simulink model "mpc_bogko"  (R2024b)
settings: Solver=VariableStepAuto  StartTime=0.0  StopTime=10  FixedStep=0.01  RelTol=1e-3
model workspace (MAT data in the model file):
  AlgnTrqCambCompl = [0 0 0 0]
  AlgnTrqSteerCompl = [0 0 0 0]
  AxlIxx = 62.3745166667
  AxlM = 160
  BumpCamber = [0 0 0 0]
  BumpCaster = [0 0 0 0]
  BumpSteer = [0 0 0 0]
  CambVsSteerAng = [0 0 0 0]
  CastVsSteerAng = [0 0 0 0]
  Cps = 2
  Cz = 5565.2246438
  CzWhlAxl = 11490.971257
  DCT_Param : object (value not decoded)
  DLCXref = [0 6.1 6.2 18 33 33.5 45 50 60]
  DLCXrefStanley1 = [0 2.4 4.8 7.2 9.6 12 17.2002368196 22.3752654753 27.5 32.6247345247 37.7997631804 43 ... (32 elements, 1x32)]
  DLCXrefStanley2 = [0 1.2 2.4 3.6 4.8 6 7.2 8.4 9.44987166868 10.0991210544 10.1 10.1008789456 ... (38 elements, 1x38)]
  DLCYref = [0 0 -5 -3.875 -3.5 1 0 0 0]
  DLCYrefStanley1 = [0 0 0 0 0 0 -0.181140468595 -0.723683795406 -1.625 -2.52631620459 -3.0688595314 -3.25 ... (32 elements, 1x32)]
  DLCYrefStanley2 = [0.1375 0.1375 0.1375 0.1375 0.1375 0.1375 0.1375 0.1375 -0.203439148031 -1.09615705337 -2.2 -3.30384294663 ... (38 elements, 1x38)]
  Downshift_Speeds = [9.5625 12.9375 16.3125 19.6875 23.0625 26.4375 29.8125 33.1875 36.5625 39.9375 43.3125 46.6875 ... (28 elements, 4x7)]
  EngRevLim = 7000
  F0z = [1067 933]
  F0zWhlAxl = 2907
  Hmax = 0.25
  Kz = 52451.0065793
  KzWhlAxl = 138031.612078
  LatCambCompl = [0 0 0 0]
  LatSteerCompl = [0 0 0 0]
  LatWhlCtrComplLat = [0 0 0 0]
  LatWhlCtrComplLngBrk = [0  0  0  0; 0  0  0  0]
  LatWhlCtrDisp = [0 0 0 0]
  LngCambCompl = [0  0  0  0; 0  0  0  0]
  LngCastCompl = [0  0  0  0; 0  0  0  0]
  LngSteerCompl = [0  0  0  0; 0  0  0  0]
  LngWhlCtrCompl = [0  0  0  0; 0  0  0  0]
  LngWhlCtrDisp = [0 0 0 0]
  MotRatios = [1 1]
  NCyl = 6
  NrmlWhlFrcOff = [2886 2886 2907 2907]
  NrmlWhlRates = [52.4510065793 52.4510065793 52.4510065793 52.4510065793]
  Pedal_Positions = [0.1 0.4 0.5 0.9]
  Pstd = 101325
  Rair = 287
  RollCamber : object (value not decoded)
  RollCaster : object (value not decoded)
  RollSteer : object (value not decoded)
  RollStiffArb = [0 0]
  RollStiffArbFrnt = 800
  RollStiffNoArb = [0 0]
  RollStiffNoArbFrnt = 0
  RollStiffNoTwstRear = 0
  ShckFrcVsCompRate = [5.5652246438 5.5652246438 5.5652246438 5.5652246438]
  Sig : Simulink.Signal (value not decoded)
  Sig1 : Simulink.Signal (value not decoded)
  StatCamber = [0 0 0 0]
  StatCaster = [0 0 0 0]
  StatLdWhlR = [0.3 0.3 0.3 0.3]
  StatToe = [0 0 0 0]
  Trans : object (value not decoded)
  Tstd = 293.15
  Upshift_Speeds = [12.9375 16.3125 19.6875 33 26.4375 29.8125 33.1875 52.5 39.9375 43.3125 46.6875 77.25 ... (28 elements, 4x7)]
  VEH : object (value not decoded)
  Vd = 0.00346
  VrtLdTrnsfr = [0 0 0 0]
  WH : Mass (value not decoded)
  dt3D = 0.05
  f_air = [0 0 0 0 0 0 0 0 0 0 0 0 ... (256 elements, 16x16)]
  f_co = [0 0 0 0 0 0 0 0 0 0 0 0 ... (256 elements, 16x16)]
  f_co2 = [0 0 0 0 0 0 0 0 0 0 0 0 ... (256 elements, 16x16)]
  f_eff = [352.135682859 352.135682859 320.724378192 303.655312657 295.930136708 291.240087194 291.240271258 291.240312459 291.240275452 291.240198499 291.240100781 291.240018769 ... (256 elements, 16x16)]
  f_fuel = [0 0 0 0 0 0 0 0 0 0 0 0 ... (256 elements, 16x16)]
  f_hc = [0 0 0 0 0 0 0 0 0 0 0 0 ... (256 elements, 16x16)]
  f_nox = [0 0 0 0 0 0 0 0 0 0 0 0 ... (256 elements, 16x16)]
  f_pm = [0 0 0 0 0 0 0 0 0 0 0 0 ... (256 elements, 16x16)]
  f_susp_axl_bp = [1 2]
  f_susp_dz_bp = [-0.325022776267 -0.315022776267 -0.305022776267 -0.205022776267 -0.105022776267 -0.00502277626717 0.0949772237328 0.194977223733 0.204977223733 0.214977223733]
  f_susp_dzdot_bp = [-3 -0.3 -0.2 -0.1 0 0.1 0.2 0.3 3]
  f_susp_fmz = [-144070.391448 -93629.24037 -75929.1118915 -20630.5828179 -15385.48216 -10140.3815021 -4895.28084414 349.819813785 -31916.3973792 18437.6709544 -83996.1993354 -33555.0482577 ... (43920 elements, 10x9x61x2x4)]
  f_susp_geom = [0 0 0 0 0 0 0 0 0 0 0 0 ... (3660 elements, 10x61x2x3)]
  f_susp_strgdelta_bp = [-0.523598775598 -0.506145483078 -0.488692190558 -0.471238898038 -0.453785605519 -0.436332312999 -0.418879020479 -0.401425727959 -0.383972435439 -0.366519142919 -0.349065850399 -0.331612557879 ... (61 elements, 1x61)]
  f_tbrake = [0 76.8593923996 105.140482948 131.533638111 157.926793274 176.658631717 176.65727296 176.656856686 176.656879077 176.657093756 176.657404516 176.65772406 ... (256 elements, 16x16)]
  f_tbrake_n_bpt = [0 649.519052838 912.419621844 1175.32019085 1438.22075986 1701.12132886 1964.02189787 2226.92246687 2489.82303588 2752.72360489 3015.62417389 3278.5247429 ... (16 elements, 1x16)]
  f_tbrake_t_bpt = [0 34.6410161514 61.0341713143 87.4273264773 113.82048164 140.213636803 166.606791966 192.999947129 219.393102292 245.786257455 272.179412618 298.572567781 ... (16 elements, 1x16)]
  f_texh = [766.752464599 766.752464599 786.17542386 801.679939032 884.591982581 910.574397722 910.571871054 910.570774534 910.570601632 910.570821151 910.571247242 910.571639815 ... (256 elements, 16x16)]
  f_twc_eff_co = [0.17 0.25 0.45 0.99 0.99 0.99 0.99]
  f_twc_eff_hc = [0.21 0.375 0.75 0.98 0.98 0.98 0.98]
  f_twc_eff_lam = [0.909090909 0.944055944 0.979020979 1 1.013986014 1.048951049 1.083916084]
  f_twc_eff_nox = [0.98 0.98 0.98 0.97 0.05 0.02 0]
  numWheel = 4
  rayDirections = [0 0 0 0 0 0 0 0 0 0 0 0 ... (363 elements, 121x3)]
  rayLengths = [20 20 20 20 20 20 20 20 20 20 20 20 ... (121 elements, 121x1)]
  rayOrigins = [0.5 0.4 0.3 0.2 0.1 0 -0.1 -0.2 -0.3 -0.4 -0.5 0.5 ... (363 elements, 121x3)]
values from neighbouring files (symbols this model uses):
  a = -2*(Cf+Cr)/(m*V)    (= -1.53333333333)    [continuousDynamics.m]    (also in getting_lqr_gain.m = -1.91273333333; mpc_simulation.m; road.m = 1.4)
  b = -1-2*(Cf*Lf-Cr*Lr)/(m*V^2)    (= -0.996444444444)    [continuousDynamics.m]    (also in getting_lqr_gain.m = -0.976308444444; mpc_simulation.m; road.m = 1.6)
  beta_road = road(:,4)    [analytic_simulation.m]    (also in lqr_simulation.m; mpc_simulation.m; plotting.m)
  c = -2*((Cf*Lf-Cr*Lr)/Jz)    (= 0.4)    [continuousDynamics.m]    (also in getting_lqr_gain.m = 2.6653; mpc_simulation.m)
  D = [0]    [getting_lqr_gain.m]    (also in mpc_simulation.m = zeros(nx,1))
  t_road = road(:,1)    [analytic_simulation.m]    (also in lqr_simulation.m; mpc_simulation.m; plotting.m; road.m = 0:dt:t_end)
  yaw_rate_road = road(:,5)    [analytic_simulation.m]    (also in lqr_simulation.m; mpc_simulation.m)
symbols that are objects in the model workspace (value not decoded): VEH
libraries: vehdynlibtire x11, vehdynlibsuspension x8, sharedtransform x6, autolibutils x5, instrumentseriallib x3, sim3dgroundtruthsensorlib x2, SignalEditorBlockLib x2, shared6dof x2, svdutilitieslib x1, vehdynlibviscommon x1, vehdynlibsteering x1, hdlsllib x1
(part 9 of 9)

== system mpc_bogko/Vehicle/Variant Subsystem/6DOF/Suspension to Chasiss Transforms/Susp2Body ==
  DCM : Inport
  VehAng : Inport  Port=2
  SuspAng : Inport  Port=3
  Fs : Inport  Port=4  Partition=on  PartitionDimension=2  PartitionWidth=1  PartitionOffset=0
  Ms : Inport  Port=5  Partition=on  PartitionDimension=2  PartitionWidth=1  PartitionOffset=0
  For Each : ForEach  DisableCoverage=on
  Inertial to Body : Product  Multiplication=Matrix(*)  InputSameDT=on  SaturateOnIntegerOverflow=on  OutDataTypeStr=Inherit: Same as first input
  Inertial to Body1 : Product  Multiplication=Matrix(*)  InputSameDT=on  SaturateOnIntegerOverflow=on  OutDataTypeStr=Inherit: Same as first input
  Reshape : Reshape
  Reshape1 : Reshape
  Rotation Angles to Direction Cosine Matrix : sharedtransform/Rotation Angles to Direction Cosine Matrix  rotationOrder=ZYX  aMode=2
  Selector : Selector  InputPortWidth=3  IndexOptions=Index vector (dialog)  Indices=[3 2 1]  OutputSizes=1
  Selector1 : Selector  InputPortWidth=3  IndexOptions=Index vector (dialog)  Indices=[1 2]  OutputSizes=1
  Selector2 : Selector  InputPortWidth=3  IndexOptions=Index vector (dialog)  Indices=[3]  OutputSizes=1
  Transpose : Math  Operator=transpose  SignedPower=on
  Unary Minus : UnaryMinus
  Vector Concatenate : Concatenate
  "transform to Inertial axes " : shared6dof/6DOF (Euler Angles)/transform to Inertial axes   SystemSampleTime=-1  VariantActivationTime=update diagram  AllowFlexibleInterface=on  Latency=0  AutoFrameSizeCalculation=off
  transform to Inertial axes 1 : shared6dof/6DOF (Euler Angles)/transform to Inertial axes   SystemSampleTime=-1  VariantActivationTime=update diagram  AllowFlexibleInterface=on  Latency=0  AutoFrameSizeCalculation=off
  FsB : Outport  ConcatenationDimension=2  VectorParamsAs1DForOutWhenUnconnected=off
  MsB : Outport  Port=2  ConcatenationDimension=2  VectorParamsAs1DForOutWhenUnconnected=off
  wires:
  Reshape/1 -> Inertial to Body/2
  Inertial to Body/1 -> FsB/1
  SuspAng/1 -> Unary Minus/1
  Selector/1 -> Rotation Angles to Direction Cosine Matrix/1
  Fs/1 -> "transform to Inertial axes "/1
  Transpose/1 -> transform to Inertial axes 1/2, "transform to Inertial axes "/2
  Rotation Angles to Direction Cosine Matrix/1 -> Transpose/1
  "transform to Inertial axes "/1 -> Reshape/1
  transform to Inertial axes 1/1 -> Reshape1/1
  Inertial to Body1/1 -> MsB/1
  Reshape1/1 -> Inertial to Body1/2
  DCM/1 -> Inertial to Body1/1, Inertial to Body/1
  Ms/1 -> transform to Inertial axes 1/1
  VehAng/1 -> Selector2/1
  Unary Minus/1 -> Selector1/1
  Selector1/1 -> Vector Concatenate/1
  Vector Concatenate/1 -> Selector/1
  Selector2/1 -> Vector Concatenate/2

== system mpc_bogko/Wheels and Tires/VDBS/Tires/Fiala Tires/Fx ==
  In1 : Inport
  In2 : Inport  Port=2
  In3 : Inport  Port=3
  In4 : Inport  Port=4
  Bus Selector{,1..3} (4 alike) : BusSelector  OutputSignals=Fx
  Vector Concatenate : Concatenate  NumInputs=4
  Out1 : Outport  VectorParamsAs1DForOutWhenUnconnected=off
  wires:
  Bus Selector3/1 -> Vector Concatenate/4  "<Fx>"
  Bus Selector2/1 -> Vector Concatenate/3  "<Fx>"
  Bus Selector1/1 -> Vector Concatenate/2  "<Fx>"
  In4/1 -> Bus Selector3/1
  In3/1 -> Bus Selector2/1
  In2/1 -> Bus Selector1/1
  Bus Selector/1 -> Vector Concatenate/1  "<Fx>"
  In1/1 -> Bus Selector/1
  Vector Concatenate/1 -> Out1/1

== system mpc_bogko/Wheels and Tires/VDBS/Tires/Fiala Tires/Fy ==
  In1 : Inport
  In2 : Inport  Port=2
  In3 : Inport  Port=3
  In4 : Inport  Port=4
  Bus Selector{,1..3} (4 alike) : BusSelector  OutputSignals=Fy
  Vector Concatenate : Concatenate  NumInputs=4
  Out1 : Outport  VectorParamsAs1DForOutWhenUnconnected=off
  wires:
  Vector Concatenate/1 -> Out1/1
  In1/1 -> Bus Selector/1
  Bus Selector/1 -> Vector Concatenate/1  "<Fy>"
  In2/1 -> Bus Selector1/1
  In3/1 -> Bus Selector2/1
  In4/1 -> Bus Selector3/1
  Bus Selector1/1 -> Vector Concatenate/2  "<Fy>"
  Bus Selector2/1 -> Vector Concatenate/3  "<Fy>"
  Bus Selector3/1 -> Vector Concatenate/4  "<Fy>"

== system mpc_bogko/Wheels and Tires/VDBS/Tires/Fiala Tires/Fz ==
  In1 : Inport
  In2 : Inport  Port=2
  In3 : Inport  Port=3
  In4 : Inport  Port=4
  Bus Selector{,1..3} (4 alike) : BusSelector  OutputSignals=Fz
  Vector Concatenate : Concatenate  NumInputs=4
  Out1 : Outport  VectorParamsAs1DForOutWhenUnconnected=off
  wires:
  Vector Concatenate/1 -> Out1/1
  In1/1 -> Bus Selector/1
  Bus Selector/1 -> Vector Concatenate/1  "<Fz>"
  In2/1 -> Bus Selector1/1
  In3/1 -> Bus Selector2/1
  In4/1 -> Bus Selector3/1
  Bus Selector1/1 -> Vector Concatenate/2  "<Fz>"
  Bus Selector2/1 -> Vector Concatenate/3  "<Fz>"
  Bus Selector3/1 -> Vector Concatenate/4  "<Fz>"

== system mpc_bogko/Wheels and Tires/VDBS/Tires/Fiala Tires/Mx ==
  In1 : Inport
  In2 : Inport  Port=2
  In3 : Inport  Port=3
  In4 : Inport  Port=4
  Bus Selector{,1..3} (4 alike) : BusSelector  OutputSignals=Mx
  Vector Concatenate : Concatenate  NumInputs=4
  Out1 : Outport  VectorParamsAs1DForOutWhenUnconnected=off
  wires:
  Vector Concatenate/1 -> Out1/1
  In1/1 -> Bus Selector/1
  Bus Selector/1 -> Vector Concatenate/1  "<Mx>"
  In2/1 -> Bus Selector1/1
  In3/1 -> Bus Selector2/1
  In4/1 -> Bus Selector3/1
  Bus Selector1/1 -> Vector Concatenate/2  "<Mx>"
  Bus Selector2/1 -> Vector Concatenate/3  "<Mx>"
  Bus Selector3/1 -> Vector Concatenate/4  "<Mx>"

== system mpc_bogko/Wheels and Tires/VDBS/Tires/Fiala Tires/My ==
  In1 : Inport
  In2 : Inport  Port=2
  In3 : Inport  Port=3
  In4 : Inport  Port=4
  Bus Selector{,1..3} (4 alike) : BusSelector  OutputSignals=My
  Vector Concatenate : Concatenate  NumInputs=4
  Out1 : Outport  VectorParamsAs1DForOutWhenUnconnected=off
  wires:
  Bus Selector3/1 -> Vector Concatenate/4  "<My>"
  Bus Selector2/1 -> Vector Concatenate/3  "<My>"
  Bus Selector1/1 -> Vector Concatenate/2  "<My>"
  In4/1 -> Bus Selector3/1
  In3/1 -> Bus Selector2/1
  In2/1 -> Bus Selector1/1
  Bus Selector/1 -> Vector Concatenate/1  "<My>"
  In1/1 -> Bus Selector/1
  Vector Concatenate/1 -> Out1/1

== system mpc_bogko/Wheels and Tires/VDBS/Tires/Fiala Tires/Mz ==
  In1 : Inport
  In2 : Inport  Port=2
  In3 : Inport  Port=3
  In4 : Inport  Port=4
  Bus Selector{,1..3} (4 alike) : BusSelector  OutputSignals=Mz
  Vector Concatenate : Concatenate  NumInputs=4
  Out1 : Outport  VectorParamsAs1DForOutWhenUnconnected=off
  wires:
  Bus Selector3/1 -> Vector Concatenate/4  "<Mz>"
  Bus Selector2/1 -> Vector Concatenate/3  "<Mz>"
  Bus Selector1/1 -> Vector Concatenate/2  "<Mz>"
  In4/1 -> Bus Selector3/1
  In3/1 -> Bus Selector2/1
  In2/1 -> Bus Selector1/1
  Bus Selector/1 -> Vector Concatenate/1  "<Mz>"
  In1/1 -> Bus Selector/1
  Vector Concatenate/1 -> Out1/1

== system mpc_bogko/Wheels and Tires/VDBS/Tires/Fiala Tires/Re ==
  In1 : Inport
  In2 : Inport  Port=2
  In3 : Inport  Port=3
  In4 : Inport  Port=4
  Bus Selector{,1..3} (4 alike) : BusSelector  OutputSignals=Re
  Vector Concatenate : Concatenate  NumInputs=4
  Out1 : Outport  VectorParamsAs1DForOutWhenUnconnected=off
  wires:
  Vector Concatenate/1 -> Out1/1
  In1/1 -> Bus Selector/1
  Bus Selector/1 -> Vector Concatenate/1  "<Re>"
  In2/1 -> Bus Selector1/1
  In3/1 -> Bus Selector2/1
  In4/1 -> Bus Selector3/1
  Bus Selector1/1 -> Vector Concatenate/2  "<Re>"
  Bus Selector2/1 -> Vector Concatenate/3  "<Re>"
  Bus Selector3/1 -> Vector Concatenate/4  "<Re>"

== system mpc_bogko/Wheels and Tires/VDBS/Tires/Fiala Tires/alpha ==
  In1 : Inport
  In2 : Inport  Port=2
  In3 : Inport  Port=3
  In4 : Inport  Port=4
  Bus Selector{,1..3} (4 alike) : BusSelector  OutputSignals=Alpha
  Vector Concatenate : Concatenate  NumInputs=4
  Out1 : Outport  VectorParamsAs1DForOutWhenUnconnected=off
  wires:
  Vector Concatenate/1 -> Out1/1
  In1/1 -> Bus Selector/1
  Bus Selector/1 -> Vector Concatenate/1  "<Alpha>"
  In2/1 -> Bus Selector1/1
  In3/1 -> Bus Selector2/1
  In4/1 -> Bus Selector3/1
  Bus Selector1/1 -> Vector Concatenate/2  "<Alpha>"
  Bus Selector2/1 -> Vector Concatenate/3  "<Alpha>"
  Bus Selector3/1 -> Vector Concatenate/4  "<Alpha>"

== system mpc_bogko/Wheels and Tires/VDBS/Tires/Fiala Tires/kappa ==
  In1 : Inport
  In2 : Inport  Port=2
  In3 : Inport  Port=3
  In4 : Inport  Port=4
  Bus Selector{,1..3} (4 alike) : BusSelector  OutputSignals=Kappa
  Vector Concatenate : Concatenate  NumInputs=4
  Out1 : Outport  VectorParamsAs1DForOutWhenUnconnected=off
  wires:
  Bus Selector3/1 -> Vector Concatenate/4  "<Kappa>"
  Bus Selector2/1 -> Vector Concatenate/3  "<Kappa>"
  Bus Selector1/1 -> Vector Concatenate/2  "<Kappa>"
  In4/1 -> Bus Selector3/1
  In3/1 -> Bus Selector2/1
  In2/1 -> Bus Selector1/1
  Bus Selector/1 -> Vector Concatenate/1  "<Kappa>"
  In1/1 -> Bus Selector/1
  Vector Concatenate/1 -> Out1/1

== system mpc_bogko/Wheels and Tires/VDBS/Tires/Fiala Tires/omega ==
  In1 : Inport
  In2 : Inport  Port=2
  In3 : Inport  Port=3
  In4 : Inport  Port=4
  Bus Selector{,1..3} (4 alike) : BusSelector  OutputSignals=Omega
  Vector Concatenate : Concatenate  NumInputs=4
  Out1 : Outport  VectorParamsAs1DForOutWhenUnconnected=off
  wires:
  In1/1 -> Bus Selector/1
  Bus Selector/1 -> Vector Concatenate/1  "<Omega>"
  In2/1 -> Bus Selector1/1
  In3/1 -> Bus Selector2/1
  In4/1 -> Bus Selector3/1
  Bus Selector1/1 -> Vector Concatenate/2  "<Omega>"
  Bus Selector2/1 -> Vector Concatenate/3  "<Omega>"
  Bus Selector3/1 -> Vector Concatenate/4  "<Omega>"
  Vector Concatenate/1 -> Out1/1

== system mpc_bogko/Wheels and Tires/VDBS/Tires/Fiala Tires/z ==
  In1 : Inport
  In2 : Inport  Port=2
  In3 : Inport  Port=3
  In4 : Inport  Port=4
  Bus Selector{,1..3} (4 alike) : BusSelector  OutputSignals=z
  Vector Concatenate : Concatenate  NumInputs=4
  Out1 : Outport  VectorParamsAs1DForOutWhenUnconnected=off
  wires:
  Bus Selector3/1 -> Vector Concatenate/4  "<z>"
  Bus Selector2/1 -> Vector Concatenate/3  "<z>"
  Bus Selector1/1 -> Vector Concatenate/2  "<z>"
  In4/1 -> Bus Selector3/1
  In3/1 -> Bus Selector2/1
  In2/1 -> Bus Selector1/1
  Bus Selector/1 -> Vector Concatenate/1  "<z>"
  In1/1 -> Bus Selector/1
  Vector Concatenate/1 -> Out1/1

== system mpc_bogko/Wheels and Tires/VDBS/Tires/Fiala Tires/zdot ==
  In1 : Inport
  In2 : Inport  Port=2
  In3 : Inport  Port=3
  In4 : Inport  Port=4
  Bus Selector{,1..3} (4 alike) : BusSelector  OutputSignals=zdot
  Vector Concatenate : Concatenate  NumInputs=4
  Out1 : Outport  VectorParamsAs1DForOutWhenUnconnected=off
  wires:
  Vector Concatenate/1 -> Out1/1
  In1/1 -> Bus Selector/1
  Bus Selector/1 -> Vector Concatenate/1  "<zdot>"
  In2/1 -> Bus Selector1/1
  In3/1 -> Bus Selector2/1
  In4/1 -> Bus Selector3/1
  Bus Selector1/1 -> Vector Concatenate/2  "<zdot>"
  Bus Selector2/1 -> Vector Concatenate/3  "<zdot>"
  Bus Selector3/1 -> Vector Concatenate/4  "<zdot>"

== system mpc_bogko/Wheels and Tires/VDBS/Tires/MF Tires/Fx ==
  In1 : Inport
  In2 : Inport  Port=2
  In3 : Inport  Port=3
  In4 : Inport  Port=4
  Bus Selector{,1..3} (4 alike) : BusSelector  OutputSignals=Fx
  Vector Concatenate : Concatenate  NumInputs=4
  Out1 : Outport  VectorParamsAs1DForOutWhenUnconnected=off
  wires:
  Bus Selector3/1 -> Vector Concatenate/4  "<Fx>"
  Bus Selector2/1 -> Vector Concatenate/3  "<Fx>"
  Bus Selector1/1 -> Vector Concatenate/2  "<Fx>"
  In4/1 -> Bus Selector3/1
  In3/1 -> Bus Selector2/1
  In2/1 -> Bus Selector1/1
  Bus Selector/1 -> Vector Concatenate/1  "<Fx>"
  In1/1 -> Bus Selector/1
  Vector Concatenate/1 -> Out1/1

== system mpc_bogko/Wheels and Tires/VDBS/Tires/MF Tires/Fy ==
  In1 : Inport
  In2 : Inport  Port=2
  In3 : Inport  Port=3
  In4 : Inport  Port=4
  Bus Selector{,1..3} (4 alike) : BusSelector  OutputSignals=Fy
  Vector Concatenate : Concatenate  NumInputs=4
  Out1 : Outport  VectorParamsAs1DForOutWhenUnconnected=off
  wires:
  Vector Concatenate/1 -> Out1/1
  In1/1 -> Bus Selector/1
  Bus Selector/1 -> Vector Concatenate/1  "<Fy>"
  In2/1 -> Bus Selector1/1
  In3/1 -> Bus Selector2/1
  In4/1 -> Bus Selector3/1
  Bus Selector1/1 -> Vector Concatenate/2  "<Fy>"
  Bus Selector2/1 -> Vector Concatenate/3  "<Fy>"
  Bus Selector3/1 -> Vector Concatenate/4  "<Fy>"

== system mpc_bogko/Wheels and Tires/VDBS/Tires/MF Tires/Fz ==
  In1 : Inport
  In2 : Inport  Port=2
  In3 : Inport  Port=3
  In4 : Inport  Port=4
  Bus Selector{,1..3} (4 alike) : BusSelector  OutputSignals=Fz
  Vector Concatenate : Concatenate  NumInputs=4
  Out1 : Outport  VectorParamsAs1DForOutWhenUnconnected=off
  wires:
  Vector Concatenate/1 -> Out1/1
  In1/1 -> Bus Selector/1
  Bus Selector/1 -> Vector Concatenate/1  "<Fz>"
  In2/1 -> Bus Selector1/1
  In3/1 -> Bus Selector2/1
  In4/1 -> Bus Selector3/1
  Bus Selector1/1 -> Vector Concatenate/2  "<Fz>"
  Bus Selector2/1 -> Vector Concatenate/3  "<Fz>"
  Bus Selector3/1 -> Vector Concatenate/4  "<Fz>"

== system mpc_bogko/Wheels and Tires/VDBS/Tires/MF Tires/Mx ==
  In1 : Inport
  In2 : Inport  Port=2
  In3 : Inport  Port=3
  In4 : Inport  Port=4
  Bus Selector{,1..3} (4 alike) : BusSelector  OutputSignals=Mx
  Vector Concatenate : Concatenate  NumInputs=4
  Out1 : Outport  VectorParamsAs1DForOutWhenUnconnected=off
  wires:
  Vector Concatenate/1 -> Out1/1
  In1/1 -> Bus Selector/1
  Bus Selector/1 -> Vector Concatenate/1  "<Mx>"
  In2/1 -> Bus Selector1/1
  In3/1 -> Bus Selector2/1
  In4/1 -> Bus Selector3/1
  Bus Selector1/1 -> Vector Concatenate/2  "<Mx>"
  Bus Selector2/1 -> Vector Concatenate/3  "<Mx>"
  Bus Selector3/1 -> Vector Concatenate/4  "<Mx>"

== system mpc_bogko/Wheels and Tires/VDBS/Tires/MF Tires/My ==
  In1 : Inport
  In2 : Inport  Port=2
  In3 : Inport  Port=3
  In4 : Inport  Port=4
  Bus Selector{,1..3} (4 alike) : BusSelector  OutputSignals=My
  Vector Concatenate : Concatenate  NumInputs=4
  Out1 : Outport  VectorParamsAs1DForOutWhenUnconnected=off
  wires:
  Bus Selector3/1 -> Vector Concatenate/4  "<My>"
  Bus Selector2/1 -> Vector Concatenate/3  "<My>"
  Bus Selector1/1 -> Vector Concatenate/2  "<My>"
  In4/1 -> Bus Selector3/1
  In3/1 -> Bus Selector2/1
  In2/1 -> Bus Selector1/1
  Bus Selector/1 -> Vector Concatenate/1  "<My>"
  In1/1 -> Bus Selector/1
  Vector Concatenate/1 -> Out1/1

== system mpc_bogko/Wheels and Tires/VDBS/Tires/MF Tires/Mz ==
  In1 : Inport
  In2 : Inport  Port=2
  In3 : Inport  Port=3
  In4 : Inport  Port=4
  Bus Selector{,1..3} (4 alike) : BusSelector  OutputSignals=Mz
  Vector Concatenate : Concatenate  NumInputs=4
  Out1 : Outport  VectorParamsAs1DForOutWhenUnconnected=off
  wires:
  Bus Selector3/1 -> Vector Concatenate/4  "<Mz>"
  Bus Selector2/1 -> Vector Concatenate/3  "<Mz>"
  Bus Selector1/1 -> Vector Concatenate/2  "<Mz>"
  In4/1 -> Bus Selector3/1
  In3/1 -> Bus Selector2/1
  In2/1 -> Bus Selector1/1
  Bus Selector/1 -> Vector Concatenate/1  "<Mz>"
  In1/1 -> Bus Selector/1
  Vector Concatenate/1 -> Out1/1

== system mpc_bogko/Wheels and Tires/VDBS/Tires/MF Tires/Re ==
  In1 : Inport
  In2 : Inport  Port=2
  In3 : Inport  Port=3
  In4 : Inport  Port=4
  Bus Selector{,1..3} (4 alike) : BusSelector  OutputSignals=Re
  Vector Concatenate : Concatenate  NumInputs=4
  Out1 : Outport  VectorParamsAs1DForOutWhenUnconnected=off
  wires:
  Vector Concatenate/1 -> Out1/1
  In1/1 -> Bus Selector/1
  Bus Selector/1 -> Vector Concatenate/1  "<Re>"
  In2/1 -> Bus Selector1/1
  In3/1 -> Bus Selector2/1
  In4/1 -> Bus Selector3/1
  Bus Selector1/1 -> Vector Concatenate/2  "<Re>"
  Bus Selector2/1 -> Vector Concatenate/3  "<Re>"
  Bus Selector3/1 -> Vector Concatenate/4  "<Re>"

== system mpc_bogko/Wheels and Tires/VDBS/Tires/MF Tires/alpha ==
  In1 : Inport
  In2 : Inport  Port=2
  In3 : Inport  Port=3
  In4 : Inport  Port=4
  Bus Selector{,1..3} (4 alike) : BusSelector  OutputSignals=Alpha
  Vector Concatenate : Concatenate  NumInputs=4
  Out1 : Outport  VectorParamsAs1DForOutWhenUnconnected=off
  wires:
  Vector Concatenate/1 -> Out1/1
  In1/1 -> Bus Selector/1
  Bus Selector/1 -> Vector Concatenate/1  "<Alpha>"
  In2/1 -> Bus Selector1/1
  In3/1 -> Bus Selector2/1
  In4/1 -> Bus Selector3/1
  Bus Selector1/1 -> Vector Concatenate/2  "<Alpha>"
  Bus Selector2/1 -> Vector Concatenate/3  "<Alpha>"
  Bus Selector3/1 -> Vector Concatenate/4  "<Alpha>"

== system mpc_bogko/Wheels and Tires/VDBS/Tires/MF Tires/kappa ==
  In1 : Inport
  In2 : Inport  Port=2
  In3 : Inport  Port=3
  In4 : Inport  Port=4
  Bus Selector{,1..3} (4 alike) : BusSelector  OutputSignals=Kappa
  Vector Concatenate : Concatenate  NumInputs=4
  Out1 : Outport  VectorParamsAs1DForOutWhenUnconnected=off
  wires:
  Bus Selector3/1 -> Vector Concatenate/4  "<Kappa>"
  Bus Selector2/1 -> Vector Concatenate/3  "<Kappa>"
  Bus Selector1/1 -> Vector Concatenate/2  "<Kappa>"
  In4/1 -> Bus Selector3/1
  In3/1 -> Bus Selector2/1
  In2/1 -> Bus Selector1/1
  Bus Selector/1 -> Vector Concatenate/1  "<Kappa>"
  In1/1 -> Bus Selector/1
  Vector Concatenate/1 -> Out1/1

== system mpc_bogko/Wheels and Tires/VDBS/Tires/MF Tires/omega ==
  In1 : Inport
  In2 : Inport  Port=2
  In3 : Inport  Port=3
  In4 : Inport  Port=4
  Bus Selector{,1..3} (4 alike) : BusSelector  OutputSignals=Omega
  Vector Concatenate : Concatenate  NumInputs=4
  Out1 : Outport  VectorParamsAs1DForOutWhenUnconnected=off
  wires:
  In1/1 -> Bus Selector/1
  Bus Selector/1 -> Vector Concatenate/1  "<Omega>"
  In2/1 -> Bus Selector1/1
  In3/1 -> Bus Selector2/1
  In4/1 -> Bus Selector3/1
  Bus Selector1/1 -> Vector Concatenate/2  "<Omega>"
  Bus Selector2/1 -> Vector Concatenate/3  "<Omega>"
  Bus Selector3/1 -> Vector Concatenate/4  "<Omega>"
  Vector Concatenate/1 -> Out1/1

== system mpc_bogko/Wheels and Tires/VDBS/Tires/MF Tires/z ==
  In1 : Inport
  In2 : Inport  Port=2
  In3 : Inport  Port=3
  In4 : Inport  Port=4
  Bus Selector{,1..3} (4 alike) : BusSelector  OutputSignals=z
  Vector Concatenate : Concatenate  NumInputs=4
  Out1 : Outport  VectorParamsAs1DForOutWhenUnconnected=off
  wires:
  Bus Selector3/1 -> Vector Concatenate/4  "<z>"
  Bus Selector2/1 -> Vector Concatenate/3  "<z>"
  Bus Selector1/1 -> Vector Concatenate/2  "<z>"
  In4/1 -> Bus Selector3/1
  In3/1 -> Bus Selector2/1
  In2/1 -> Bus Selector1/1
  Bus Selector/1 -> Vector Concatenate/1  "<z>"
  In1/1 -> Bus Selector/1
  Vector Concatenate/1 -> Out1/1

== system mpc_bogko/Wheels and Tires/VDBS/Tires/MF Tires/zdot ==
  In1 : Inport
  In2 : Inport  Port=2
  In3 : Inport  Port=3
  In4 : Inport  Port=4
  Bus Selector{,1..3} (4 alike) : BusSelector  OutputSignals=zdot
  Vector Concatenate : Concatenate  NumInputs=4
  Out1 : Outport  VectorParamsAs1DForOutWhenUnconnected=off
  wires:
  Vector Concatenate/1 -> Out1/1
  In1/1 -> Bus Selector/1
  Bus Selector/1 -> Vector Concatenate/1  "<zdot>"
  In2/1 -> Bus Selector1/1
  In3/1 -> Bus Selector2/1
  In4/1 -> Bus Selector3/1
  Bus Selector1/1 -> Vector Concatenate/2  "<zdot>"
  Bus Selector2/1 -> Vector Concatenate/3  "<zdot>"
  Bus Selector3/1 -> Vector Concatenate/4  "<zdot>"

== system mpc_bogko/Environment/Ground Feedback/3D Engine/3D Engine Source/Multiple Points/For Each Subsystem ==
  phi,theta,psi : Inport  Partition=on  PartitionDimension=2  PartitionWidth=1  PartitionOffset=0
  For Each : ForEach  DisableCoverage=on
  Rotation Angles to Direction Cosine Matrix1 : sharedtransform/Rotation Angles to Direction Cosine Matrix  rotationOrder=YXZ  aMode=2
  Selector5 : Selector  InputPortWidth=3  IndexOptions=Index vector (dialog)  Indices=[2 1 3]  OutputSizes=1
  WheelDCM : Outport  ConcatenationDimension=3
  wires:
  Selector5/1 -> Rotation Angles to Direction Cosine Matrix1/1
  Rotation Angles to Direction Cosine Matrix1/1 -> WheelDCM/1
  phi,theta,psi/1 -> Selector5/1

== matlab function mpc_bogko/Vehicle/Variant Subsystem/6DOF/Suspension to Chasiss Transforms/Estimated Unsprung Mass Orientation ==
  data: angles output size=3; angleIn input size=3; GeomXYZ output size=3; GemoXYZIn input size=3; Ground input size=4; trackW parameter; wheelB parameter
function [angles,GeomXYZ]= three26(angleIn, GemoXYZIn, Ground,trackW, wheelB)%#codegen
coder.allowpcode('plain')
% Copyright 2018 The MathWorks, Inc.
[angles,GeomXYZ]= vdynthree2six(angleIn, GemoXYZIn, Ground,trackW, wheelB);

== matlab function mpc_bogko/Wheels and Tires/VDBS/Veh2Tire/Camber Angle ==
  data: u input; y output
function y = fcn(u)
temp = squeeze(u(3,2:3,:));
y=atan(temp(1,:)./temp(2,:))';

== matlab function mpc_bogko/LQR Controller/u=-k*e/gain ==
  data: V input; k1 output; k2 output
function [k1,k2]= gain_scheduling(V)


Ve=[
0.200000 0.121576 48.390226;
0.400000 0.352582 96.752944;
0.600000 0.737210 145.083666;
0.800000 1.274885 193.363623;
1.000000 1.964809 241.575549;
1.200000 2.805959 289.702568;
1.400000 3.797097 337.728069;
1.600000 4.936770 385.635703;
1.800000 6.223321 433.409408;
2.000000 7.654893 481.033432;
2.200000 9.229437 528.492366;
2.400000 10.944722 575.771175;
2.600000 12.798342 622.855223;
2.800000 14.787729 669.730298;
3.000000 16.910159 716.382638;
3.200000 19.162765 762.798953;
3.400000 21.542547 808.966441;
3.600000 24.046383 854.872805;
3.800000 26.671041 900.506270;
4.000000 29.413188 945.855591;
4.200000 32.269405 990.910066;
4.400000 35.236193 1035.659538;
4.600000 38.309987 1080.094404;
4.800000 41.487170 1124.205617;
5.000000 44.764077 1167.984684;
5.200000 48.137009 1211.423665;
5.400000 51.602243 1254.515172;
5.600000 55.156040 1297.252362;
5.800000 58.794659 1339.628927;
6.000000 62.514357 1381.639093;
6.200000 66.311406 1423.277603;
6.400000 70.182095 1464.539710;
6.600000 74.122741 1505.421163;
6.800000 78.129695 1545.918196;
7.000000 82.199345 1586.027513;
7.200000 86.328128 1625.746271;
7.400000 90.512531 1665.072070;
7.600000 94.749097 1704.002932;
7.800000 99.034429 1742.537288;
8.000000 103.365195 1780.673963;
8.200000 107.738132 1818.412153;
8.400000 112.150046 1855.751416;
8.600000 116.597819 1892.691651;
8.800000 121.078407 1929.233082;
9.000000 125.588848 1965.376242;
9.200000 130.126254 2001.121956;
9.400000 134.687823 2036.471327;
9.600000 139.270831 2071.425717;
9.800000 143.872639 2105.986733;
10.000000 148.490690 2140.156214;
10.200000 153.122509 2173.936213;
10.400000 157.765704 2207.328982;
10.600000 162.417966 2240.336964;
10.800000 167.077067 2272.962774;
11.000000 171.740860 2305.209186;
11.200000 176.407280 2337.079126;
11.400000 181.074338 2368.575653;
11.600000 185.740124 2399.701954;
11.800000 190.402806 2430.461328;
12.000000 195.060626 2460.857177;
12.200000 199.711900 2490.892999;
12.400000 204.355016 2520.572373;
12.600000 208.988433 2549.898954;
12.800000 213.610679 2578.876465;
13.000000 218.220348 2607.508685;
13.200000 222.816100 2635.799443;
13.400000 227.396661 2663.752614;
13.600000 231.960816 2691.372105;
13.800000 236.507411 2718.661856;
14.000000 241.035352 2745.625829;
14.200000 245.543598 2772.268006;
14.400000 250.031167 2798.592379;
14.600000 254.497128 2824.602948;
14.800000 258.940600 2850.303717;
15.000000 263.360754 2875.698688;
15.200000 267.756807 2900.791856;
15.400000 272.128023 2925.587209;
15.600000 276.473710 2950.088720;
15.800000 280.793221 2974.300347;
16.000000 285.085946 2998.226027;
16.200000 289.351319 3021.869678;
16.400000 293.588810 3045.235191;
16.600000 297.797926 3068.326430;
16.800000 301.978209 3091.147232;
17.000000 306.129236 3113.701401;
17.200000 310.250616 3135.992709;
17.400000 314.341988 3158.024893;
17.600000 318.403023 3179.801656;
17.800000 322.433418 3201.326662;
18.000000 326.432901 3222.603537;
18.200000 330.401222 3243.635869;
18.400000 334.338159 3264.427202;
18.600000 338.243514 3284.981044;
18.800000 342.117110 3305.300858;
19.000000 345.958794 3325.390065;
19.200000 349.768432 3345.252044;
19.400000 353.545911 3364.890131;
19.600000 357.291138 3384.307616;
19.800000 361.004036 3403.507749;
20.000000 364.684546 3422.493733



];
k1=0; k2=0;
    for j = 1:100
        if Ve(j,1) < V
            continue
        else
            k1 = Ve(j,2);
            k2 = Ve(j,3);
            break
        end
    end

end

== matlab function mpc_bogko/LQR Controller/u=-k*e/gain_2 ==
  data: V input; k1 output; k2 output
function [k1,k2]= gain_scheduling(V)


Ve=[
0.200000 23.936091 9589.473950;
0.400000 65.811325 18678.808216;
0.600000 126.741055 26924.306247;
0.800000 198.022190 34180.035636;
1.000000 272.629837 40455.344773;
1.200000 345.939154 45842.880831;
1.400000 415.356343 50464.193341;
1.600000 479.673124 54440.000831;
1.800000 538.517188 57877.678927;
2.000000 591.976913 60867.917563;
2.200000 640.370963 63485.439607;
2.400000 684.115602 65791.153362;
2.600000 723.652003 67834.555555;
2.800000 759.408624 69655.921878;
3.000000 791.783394 71288.148388;
3.200000 821.136808 72758.241543;
3.400000 847.790799 74088.501945;
3.600000 872.030511 75297.457235;
3.800000 894.107397 76400.595660;
4.000000 914.242749 77410.943604;
4.200000 932.631238 78339.521751;
4.400000 949.444216 79195.706990;
4.600000 964.832712 79987.521020;
4.800000 978.930075 80721.861786;
5.000000 991.854293 81404.690113;
5.200000 1003.709991 82041.181083;
5.400000 1014.590173 82635.847509;
5.600000 1024.577708 83192.641197;
5.800000 1033.746619 83715.036455;
6.000000 1042.163185 84206.099304;
6.200000 1049.886895 84668.545131;
6.400000 1056.971271 85104.786956;
6.600000 1063.464576 85516.976011;
6.800000 1069.410428 85907.036016;
7.000000 1074.848335 86276.692257;
7.200000 1079.814155 86627.496351;
7.400000 1084.340504 86960.847413;
7.600000 1088.457103 87278.010229;
7.800000 1092.191092 87580.130907;
8.000000 1095.567296 87868.250398;
8.200000 1098.608465 88143.316228;
8.400000 1101.335485 88406.192693;
8.600000 1103.767559 88657.669763;
8.800000 1105.922374 88898.470865;
9.000000 1107.816245 89129.259719;
9.200000 1109.464246 89350.646345;
9.400000 1110.880323 89563.192369;
9.600000 1112.077394 89767.415711;
9.800000 1113.067449 89963.794739;
10.000000 1113.861621 90152.771961;
10.200000 1114.470271 90334.757316;
10.400000 1114.903044 90510.131105;
10.600000 1115.168937 90679.246614;
10.800000 1115.276346 90842.432464;
11.000000 1115.233120 90999.994725;
11.200000 1115.046601 91152.218805;
11.400000 1114.723666 91299.371168;
11.600000 1114.270763 91441.700873;
11.800000 1113.693943 91579.440967;
12.000000 1112.998890 91712.809753;
12.200000 1112.190949 91842.011933;
12.400000 1111.275151 91967.239647;
12.600000 1110.256232 92088.673425;
12.800000 1109.138662 92206.483044;
13.000000 1107.926655 92320.828319;
13.200000 1106.624191 92431.859820;
13.400000 1105.235034 92539.719530;
13.600000 1103.762741 92644.541450;
13.800000 1102.210680 92746.452146;
14.000000 1100.582043 92845.571263;
14.200000 1098.879853 92942.011984;
14.400000 1097.106980 93035.881467;
14.600000 1095.266147 93127.281237;
14.800000 1093.359940 93216.307547;
15.000000 1091.390818 93303.051722;
15.200000 1089.361120 93387.600467;
15.400000 1087.273071 93470.036152;
15.600000 1085.128791 93550.437086;
15.800000 1082.930297 93628.877759;
16.000000 1080.679516 93705.429070;
16.200000 1078.378284 93780.158548;
16.400000 1076.028353 93853.130543;
16.600000 1073.631396 93924.406411;
16.800000 1071.189013 93994.044692;
17.000000 1068.702732 94062.101261;
17.200000 1066.174015 94128.629484;
17.400000 1063.604261 94193.680357;
17.600000 1060.994809 94257.302631;
17.800000 1058.346942 94319.542939;
18.000000 1055.661888 94380.445908;
18.200000 1052.940827 94440.054265;
18.400000 1050.184888 94498.408938;
18.600000 1047.395155 94555.549150;
18.800000 1044.572670 94611.512503;
19.000000 1041.718433 94666.335068;
19.200000 1038.833403 94720.051454;
19.400000 1035.918505 94772.694888;
19.600000 1032.974624 94824.297278;
19.800000 1030.002616 94874.889282;
20.000000 1027.003301 94924.500367



];
k1=0; k2=0;
    for j = 1:100
        if Ve(j,1) < V
            continue
        else
            k1 = Ve(j,2);
            k2 = Ve(j,3);
            break
        end
    end

end

== matlab function mpc_bogko/LQR Controller/u=-k*e/gain_1 ==
  data: V input; k1 output; k2 output
function [k1,k2]= gain_scheduling(V)


Ve=[
0.200000 2.427818 966.944704;
0.400000 7.002986 1928.223778;
0.600000 14.510193 2878.833766;
0.800000 24.780921 3813.869810;
1.000000 37.595205 4728.988559;
1.200000 52.694991 5620.488119;
1.400000 69.798260 6485.359404;
1.600000 88.612528 7321.294698;
1.800000 108.846685 8126.659059;
2.000000 130.220563 8900.434039;
2.200000 152.472004 9642.143879;
2.400000 175.361539 10351.773329;
2.600000 198.674956 11029.684434;
2.800000 222.224173 11676.537534;
3.000000 245.846816 12293.219776;
3.200000 269.404914 12880.782848;
3.400000 292.783012 13440.390399;
3.600000 315.885995 13973.274867;
3.800000 338.636787 14480.702898;
4.000000 360.974083 14963.948301;
4.200000 382.850196 15424.271453;
4.400000 404.229072 15862.904025;
4.600000 425.084492 16281.038070;
4.800000 445.398493 16679.818569;
5.000000 465.159970 17060.338719;
5.200000 484.363473 17423.637314;
5.400000 503.008180 17770.697734;
5.600000 521.097009 18102.448124;
5.800000 538.635880 18419.762440;
6.000000 555.633087 18723.462109;
6.200000 572.098772 19014.318103;
6.400000 588.044490 19293.053283;
6.600000 603.482847 19560.344883;
6.800000 618.427199 19816.827067;
7.000000 632.891409 20063.093481;
7.200000 646.889643 20299.699761;
7.400000 660.436213 20527.165967;
7.600000 673.545438 20745.978914;
7.800000 686.231545 20956.594396;
8.000000 698.508582 21159.439288;
8.200000 710.390355 21354.913525;
8.400000 721.890376 21543.391961;
8.600000 733.021827 21725.226102;
8.800000 743.797532 21900.745732;
9.000000 754.229936 22070.260415;
9.200000 764.331095 22234.060902;
9.400000 774.112666 22392.420430;
9.600000 783.585910 22545.595933;
9.800000 792.761685 22693.829158;
10.000000 801.650456 22837.347705;
10.200000 810.262302 22976.365988;
10.400000 818.606916 23111.086124;
10.600000 826.693625 23241.698759;
10.800000 834.531392 23368.383831;
11.000000 842.128828 23491.311279;
11.200000 849.494209 23610.641694;
11.400000 856.635481 23726.526932;
11.600000 863.560274 23839.110676;
11.800000 870.275915 23948.528956;
12.000000 876.789439 24054.910636;
12.200000 883.107600 24158.377863;
12.400000 889.236882 24259.046487;
12.600000 895.183512 24357.026448;
12.800000 900.953467 24452.422135;
13.000000 906.552491 24545.332727;
13.200000 911.986096 24635.852500;
13.400000 917.259579 24724.071123;
13.600000 922.378031 24810.073927;
13.800000 927.346339 24893.942158;
14.000000 932.169204 24975.753213;
14.200000 936.851143 25055.580860;
14.400000 941.396499 25133.495445;
14.600000 945.809449 25209.564083;
14.800000 950.094008 25283.850838;
15.000000 954.254043 25356.416891;
15.200000 958.293272 25427.320698;
15.400000 962.215274 25496.618135;
15.600000 966.023496 25564.362640;
15.800000 969.721256 25630.605340;
16.000000 973.311749 25695.395174;
16.200000 976.798057 25758.779004;
16.400000 980.183145 25820.801726;
16.600000 983.469875 25881.506368;
16.800000 986.661004 25940.934187;
17.000000 989.759191 25999.124754;
17.200000 992.767003 26056.116045;
17.400000 995.686914 26111.944510;
17.600000 998.521314 26166.645157;
17.800000 1001.272508 26220.251617;
18.000000 1003.942723 26272.796210;
18.200000 1006.534110 26324.310010;
18.400000 1009.048746 26374.822901;
18.600000 1011.488639 26424.363635;
18.800000 1013.855728 26472.959883;
19.000000 1016.151890 26520.638288;
19.200000 1018.378938 26567.424505;
19.400000 1020.538625 26613.343255;
19.600000 1022.632650 26658.418357;
19.800000 1024.662654 26702.672778;
20.000000 1026.630227 26746.128662


];
k1=0; k2=0;
    for j = 1:100
        if Ve(j,1) < V
            continue
        else
            k1 = Ve(j,2);
            k2 = Ve(j,3);
            break
        end
    end

end

== matlab function mpc_bogko/LQR Controller/u=-k*e/gain_3 ==
  data: V input; k1 output; k2 output
function [k1,k2]= gain_scheduling(V)


Ve=[
0.200000 211.295941 89099.626162;
0.400000 430.474881 149992.378964;
0.600000 616.465946 187846.971108;
0.800000 753.833305 212405.251228;
1.000000 853.730170 229328.929229;
1.200000 927.171251 241609.941963;
1.400000 981.925603 250895.940800;
1.600000 1023.204912 258149.953328;
1.800000 1054.527558 263966.885250;
2.000000 1078.319138 268732.111440;
2.200000 1096.292516 272705.483009;
2.400000 1109.685822 276068.247242;
2.600000 1119.413521 278950.519639;
2.800000 1126.164304 281448.046375;
3.000000 1130.465984 283632.806473;
3.200000 1132.729470 285559.931605;
3.400000 1133.279201 287272.348793;
3.600000 1132.374608 288803.972155;
3.800000 1130.225537 290181.945181;
4.000000 1127.003493 291428.246715;
4.200000 1122.849983 292560.861387;
4.400000 1117.882773 293594.646076;
4.600000 1112.200652 294541.980549;
4.800000 1105.887093 295413.262387;
5.000000 1099.013104 296217.287964;
5.200000 1091.639466 296961.548911;
5.400000 1083.818505 297652.465126;
5.600000 1075.595511 298295.569630;
5.800000 1067.009880 298895.656464;
6.000000 1058.096042 299456.899977;
6.200000 1048.884215 299982.951741;
6.400000 1039.401034 300477.019848;
6.600000 1029.670063 300941.934208;
6.800000 1019.712228 301380.200642;
7.000000 1009.546170 301794.045962;
7.200000 999.188556 302185.455727;
7.400000 988.654328 302556.206037;
7.600000 977.956921 302907.890432;
7.800000 967.108452 303241.942746;
8.000000 956.119874 303559.656618;
8.200000 945.001113 303862.202211;
8.400000 933.761188 304150.640594;
8.600000 922.408310 304425.936162;
8.800000 910.949972 304688.967393;
9.000000 899.393025 304940.536212;
9.200000 887.743745 305181.376139;
9.400000 876.007893 305412.159437;
9.600000 864.190769 305633.503368;
9.800000 852.297252 305845.975708;
10.000000 840.331845 306050.099604;
10.200000 828.298711 306246.357872;
10.400000 816.201702 306435.196815;
10.600000 804.044390 306617.029604;
10.800000 791.830090 306792.239297;
11.000000 779.561883 306961.181536;
11.200000 767.242640 307124.186951;
11.400000 754.875034 307281.563325;
11.600000 742.461561 307433.597529;
11.800000 730.004553 307580.557273;
12.000000 717.506191 307722.692675;
12.200000 704.968518 307860.237685;
12.400000 692.393450 307993.411369;
12.600000 679.782784 308122.419074;
12.800000 667.138209 308247.453486;
13.000000 654.461314 308368.695591;
13.200000 641.753593 308486.315548;
13.400000 629.016455 308600.473489;
13.600000 616.251229 308711.320243;
13.800000 603.459170 308818.998006;
14.000000 590.641462 308923.640947;
14.200000 577.799225 309025.375769;
14.400000 564.933521 309124.322218;
14.600000 552.045352 309220.593556;
14.800000 539.135672 309314.296993;
15.000000 526.205383 309405.534088;
15.200000 513.255343 309494.401112;
15.400000 500.286365 309580.989393;
15.600000 487.299223 309665.385626;
15.800000 474.294655 309747.672163;
16.000000 461.273361 309827.927283;
16.200000 448.236009 309906.225439;
16.400000 435.183235 309982.637492;
16.600000 422.115646 310057.230921;
16.800000 409.033823 310130.070024;
17.000000 395.938318 310201.216106;
17.200000 382.829660 310270.727646;
17.400000 369.708354 310338.660462;
17.600000 356.574884 310405.067860;
17.800000 343.429714 310470.000770;
18.000000 330.273286 310533.507883;
18.200000 317.106025 310595.635769;
18.400000 303.928339 310656.428990;
18.600000 290.740618 310715.930212;
18.800000 277.543237 310774.180298;
19.000000 264.336557 310831.218409;
19.200000 251.120922 310887.082087;
19.400000 237.896666 310941.807340;
19.600000 224.664108 310995.428719;
19.800000 211.423556 311047.979389;
20.000000 198.175305 311099.491204


];
k1=0; k2=0;
    for j = 1:100
        if Ve(j,1) < V
            continue
        else
            k1 = Ve(j,2);
            k2 = Ve(j,3);
            break
        end
    end

end
